simulink model "Converter2_Combined"  (R2025a)
settings: Solver=ode15s  StartTime=0.0  StopTime=10  MaxStep=1e-4  RelTol=1e-4  EnableMultiTasking=on
libraries: spsCurrentMeasurementLib x5, spsSeriesRLCBranchLib x5, spsDCVoltageSourceLib x2, slpidlib x2, spsPWMGenerator2LevelLib x2, spsMosfetLib x2, simulink x2, spsVoltageMeasurementLib x2, spsControlledCurrentSourceLib x1, spsFirstOrderFilterLib x1, spsGroundLib x1, spspowerguiLib x1
settings Model: SimulationMode=accelerator  Creator=The MathWorks, Inc.  LastModifiedBy=kaust
settings SolverCC: MaxOrder=4.0  ZeroCrossAlgorithm=Adaptive
settings DataIOCC: LimitDataPoints=on  SaveFormat=Array  SaveOutput=off  SignalLogging=off  SaveTime=off  ReturnWorkspaceOutputs=off
settings OptimizationCC: ExpressionDepthLimit=2147483647.0  LifeSpan=inf
settings DebuggingCC: UnderspecifiedInitializationDetection=Classic  MergeDetectMultiDrivingBlocksExec=none  IgnoredZcDiagnostic=none  SolverPrmCheckMsg=warning  FcnCallInpInsideContextMsg=warning  UnconnectedInputMsg=warning  UnconnectedOutputMsg=warning  UnconnectedLineMsg=warning  StateNameClashWarn=warning  SFUnexpectedBacktrackingDiag=warning  SFNoUnconditionalDefaultTransitionDiag=warning  SFExecutionAtInitializationDiag=none  ArithmeticOperatorsInVariantConditions=warning
settings HardwareCC: ProdBitPerPointer=32.0  ProdBitPerSizeT=32.0  ProdBitPerPtrDiffT=32.0  ProdLargestAtomicFloat=None  ProdIntDivRoundTo=Undefined  ProdEndianess=Unspecified  ProdWordSize=32.0  ProdHWDeviceType=32-bit Generic
settings ModelReferenceCC: EnableRefExpFcnMdlSchedulingChecks=on  PropagateSignalLabelsOutOfModel=off
settings SFSimCC: SimUseLocalCustomCode=off  CustomCodeUndefinedFunction=UseInterfaceOnly
settings RTWCC: RTWUseLocalCustomCode=off  GPUComputeCapability=3.5  DLArmComputeVersion=19.05
settings CodeAppCC: StateflowObjectComments=on
settings GRTTargetCC: TargetLangStandard=C89/C90 (ANSI)  CombineOutputUpdateFcns=off  GRTInterface=on
settings ConfigComp: CovMetricSettings=dw  CovSaveCumulativeToWorkspaceVar=on  CovSaveSingleToWorkspaceVar=on  CovExternalEMLEnable=off  CovSFcnEnable=off
settings SimscapeCC: SimscapeNormalizeSystem=off  SimscapeNominalValues={1, 'bar'; 1, 'cm^3/s'; 1, 'bar*kg/s'; 1, 'kJ/kg'; 1, 'kW'; }

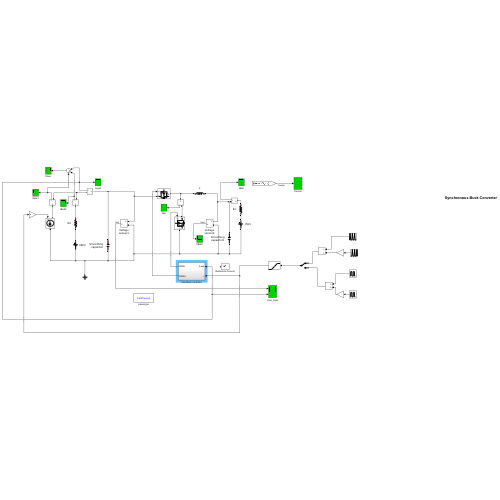
[thumbnail: Simulink's stored preview of the top-level diagram]
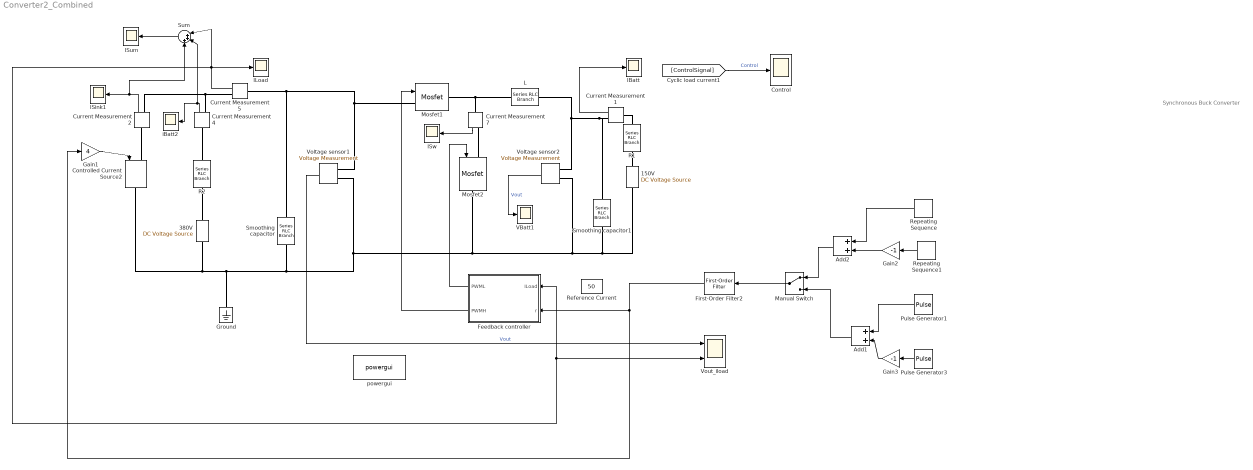
== system Converter2_Combined ==
  note: Synchronous Buck Converter
  150V : spsDCVoltageSourceLib/DC Voltage Source  Amplitude=150  Measurements=None
  380V : spsDCVoltageSourceLib/DC Voltage Source  Amplitude=380  Measurements=None
  Add1 : Sum
  Add2 : Sum
  Control : Scope
      settings: TimeSpan=0.01  ActiveDisplayYMinimum=-0.0024647053532001208  ActiveDisplayYMaximum=0.023182348178801094  DataLoggingVariableName=Control  DataLoggingSaveFormat=Array
  Controlled Current Source2 : spsControlledCurrentSourceLib/Controlled Current Source  Initialize=on  Source_Type=AC  Amplitude=0  Phase=0  Frequency=0  Measurements=None
  Current Measurement{1..2,4..5,7} (5 alike) : spsCurrentMeasurementLib/Current Measurement  PhasorSimulation=off  OutputType=Complex  PSBequivalent=0
  Feedback controller : Subsystem
  First-Order Filter2 : spsFirstOrderFilterLib/First-Order Filter  FilterType=Lowpass  Tc=5e-3  Ts=0  Initialize=off  Vac_Init=[0, 0, 60]  Vdc_Init=0  PlotResponse=off  FreqRange="[0,  200,  1]"
  Gain1 : Gain  Gain=4
  Gain2 : Gain  Gain=-1
  Gain3 : Gain  Gain=-1
  Ground : spsGroundLib/Ground  LConnTagsString=a
  IBatt : Scope
      settings: TimeSpan=0.01  ActiveDisplayYMinimum=-4410.7984256590225  ActiveDisplayYMaximum=16926.559366246598  DataLoggingVariableName=Isrc_sps1  DataLoggingSaveFormat=Array
  ILoad : Scope
      settings: TimeSpan=0.01  ActiveDisplayYMinimum=-119.68929460234355  ActiveDisplayYMaximum=1093.0850139818504  DataLoggingVariableName=Isrc_sps  DataLoggingSaveFormat=Array
  ISink1 : Scope
      settings: TimeSpan=0.01  ActiveDisplayYMinimum=-12.499999999999996  ActiveDisplayYMaximum=112.5  DataLoggingVariableName=Isrc_sps3  DataLoggingSaveFormat=Array
  ISum : Scope
      settings: TimeSpan=0.01  ActiveDisplayYMinimum=-1.7763568394002505E-14  ActiveDisplayYMaximum=1.7763568394002505E-14  DataLoggingVariableName=Isrc_sps4  DataLoggingSaveFormat=Array
  ISw : Scope
      settings: TimeSpan=0.01  ActiveDisplayYMinimum=-4410.7984256590225  ActiveDisplayYMaximum=16926.559366246598  DataLoggingVariableName=Isrc_sps6  DataLoggingSaveFormat=Array
  L : spsSeriesRLCBranchLib/Series RLC Branch  LConnTagsString=__new0  RConnTagsString=__new0  BranchType=L  Resistance=15  Inductance=1e-06  SetiL0=off  InitialCurrent=0  Capacitance=1e-6  Setx0=off  InitialVoltage=0  Measurements=None
  Manual Switch : ManualSwitch
  Mosfet1 : spsMosfetLib/Mosfet  Ron=0.1  Lon=0  Rd=0.01  Vfd=0.8  IC=0  Rs=1e5  Cs=inf  Measurements=off
  Mosfet2 : spsMosfetLib/Mosfet  Ron=0.1  Lon=0  Rd=0.01  Vfd=0.8  IC=0  Rs=1e4  Cs=inf  Measurements=off
  Pulse Generator1 : DiscretePulseGenerator  PulseType=Time based  Amplitude=50  Period=0.5  PulseWidth=50
  Pulse Generator3 : DiscretePulseGenerator  PulseType=Time based  Amplitude=50  Period=0.5  PulseWidth=50  PhaseDelay=0.25
  R1 : spsSeriesRLCBranchLib/Series RLC Branch  LConnTagsString=__new0  RConnTagsString=__new0  BranchType=R  Resistance=0.01  Inductance=1e-3  SetiL0=off  InitialCurrent=0  Capacitance=1e-6  Setx0=off  InitialVoltage=0  Measurements=None
  R2 : spsSeriesRLCBranchLib/Series RLC Branch  LConnTagsString=__new0  RConnTagsString=__new0  BranchType=R  Resistance=0.01  Inductance=1e-3  SetiL0=off  InitialCurrent=0  Capacitance=1e-6  Setx0=off  InitialVoltage=0  Measurements=None
  Reference Current : Constant  Value=50
  Repeating Sequence : simulink/Sources/Repeating Sequence  rep_seq_t=[0 0.25 0.5 0.75 1 ]  rep_seq_y=[0 50 0 0 0]
  Repeating Sequence1 : simulink/Sources/Repeating Sequence  rep_seq_t=[0 0.25 0.5 0.75 1 ]  rep_seq_y=[0 0 0 50 0]
  Smoothing capacitor : spsSeriesRLCBranchLib/Series RLC Branch  LConnTagsString=__new0  RConnTagsString=__new0  BranchType=C  Resistance=1  Inductance=1e-3  SetiL0=off  InitialCurrent=0  Capacitance=10e-3  Setx0=off  InitialVoltage=0  Measurements=None
  Smoothing capacitor1 : spsSeriesRLCBranchLib/Series RLC Branch  LConnTagsString=__new0  RConnTagsString=__new0  BranchType=C  Resistance=1  Inductance=1e-3  SetiL0=off  InitialCurrent=0  Capacitance=10e-3  Setx0=off  InitialVoltage=0  Measurements=None
  Sum : Sum  Inputs=|+++
  VBatt1 : Scope
      settings: TimeSpan=0.01  ActiveDisplayYMinimum=-4410.7984256590225  ActiveDisplayYMaximum=16926.559366246598  DataLoggingVariableName=Isrc_sps5  DataLoggingSaveFormat=Array
  Voltage sensor1 : spsVoltageMeasurementLib/Voltage Measurement  PhasorSimulation=off  OutputType=Complex  PSBequivalent=0
  Voltage sensor2 : spsVoltageMeasurementLib/Voltage Measurement  PhasorSimulation=off  OutputType=Complex  PSBequivalent=0
  Vout_iload : Scope  NumInputPorts=2
      settings: TimeSpan=0.01  ActiveDisplayYMinimum=376.83408924703053  ActiveDisplayYMaximum=382.12539978082276  DataLoggingVariableName=Vout_sps  DataLoggingSaveFormat=Array
  iBatt2 : Scope
      settings: TimeSpan=0.01  ActiveDisplayYMinimum=-212.44166562760256  ActiveDisplayYMaximum=295.23155792169746  DataLoggingVariableName=Isrc_sps2  DataLoggingSaveFormat=Array
  powergui : spspowerguiLib/powergui  Priority=1  SimulationMode=Continuous  SampleTime=50e-6  frequency=60  Iterations=50  frequencyindice=0  Pbase=100e6  ErrMax=1e-4  UnitsV=kV  UnitsW=MW  buscounter=0  FunctionMessages=off  echomessages=off  EnableUseOfTLC=off  CurrentSourceSwitches=off  DisableSnubberDevices=off  DisableRonSwitches=off  DisableVfSwitches=off  DisplayEquations=off  AutomaticDiscreteSolvers=off  SolverType=Tustin/Backward Euler (TBE)  Interpol=off  ExternalGateDelay=off  methode=off  Ts=100  x0status=blocks  SPID=on  SwTol=0  HookPort=off  NonlinearTolerance=1e-4  nMaxIteration=100  ContinueOnMaxIteration=off  RestoreLinks=warning  ResistiveCurrentMeasurement=off  Frange=[0:2:500]  Ylog=off  Xlog=on  ShowGrid=off  save=off  variable=ZData  structure=0  ZoomFFT=on  StartTime=0.0  cycles=1  DisplayStyle=1  fundamental=60  FreqAxis=off  MaxFrequency=1000  frequencyindicesteady=1  RmsSteady=1  display=off
  wires:
  Feedback controller/1(PWML) -> Mosfet2/1
  [ControlSignal] -> Control/1  "Control"
  Current Measurement5/1 -> Sum/1, ILoad/1, Feedback controller/1(ILoad), Vout_iload/2
  Feedback controller/2(PWMH) -> Mosfet1/1
  Voltage sensor1/1 -> Vout_iload/1  "Vout"
  Current Measurement1/1 -> IBatt/1
  Current Measurement4/1 -> iBatt2/1, Sum/2
  Current Measurement2/1 -> Sum/3, ISink1/1
  Sum/1 -> ISum/1
  Voltage sensor2/1 -> VBatt1/1  "Vout"
  Current Measurement7/1 -> ISw/1
  First-Order Filter2/1 -> Feedback controller/2(r), Gain1/1
  Gain1/1 -> Controlled Current Source2/1
  Repeating Sequence/1 -> Add2/1
  Repeating Sequence1/1 -> Gain2/1
  Gain2/1 -> Add2/2
  Add2/1 -> Manual Switch/1
  Manual Switch/1 -> First-Order Filter2/1
  Gain3/1 -> Add1/2
  Add1/1 -> Manual Switch/2
  Pulse Generator1/1 -> Add1/1
  Pulse Generator3/1 -> Gain3/1
  connections:
  Mosfet2/RConn1 -- Smoothing capacitor/RConn1 -- Controlled Current Source2/RConn1 -- 380V/LConn1 -- Ground/LConn1 -- Voltage sensor1/LConn2 -- Smoothing capacitor1/RConn1 -- 150V/LConn1 -- Voltage sensor2/LConn2
  L/RConn1 -- Smoothing capacitor1/LConn1 -- Current Measurement1/RConn1 -- Voltage sensor2/LConn1
  L/LConn1 -- Current Measurement7/LConn1 -- Mosfet1/RConn1
  Smoothing capacitor/LConn1 -- Voltage sensor1/LConn1 -- Mosfet1/LConn1 -- Current Measurement5/LConn1
  150V/RConn1 -- R1/RConn1
  Current Measurement5/RConn1 -- Current Measurement2/RConn1 -- Current Measurement4/RConn1
  Current Measurement2/LConn1 -- Controlled Current Source2/LConn1
  380V/RConn1 -- R2/RConn1
  Current Measurement4/LConn1 -- R2/LConn1
  R1/LConn1 -- Current Measurement1/LConn1
  Current Measurement7/RConn1 -- Mosfet2/LConn1

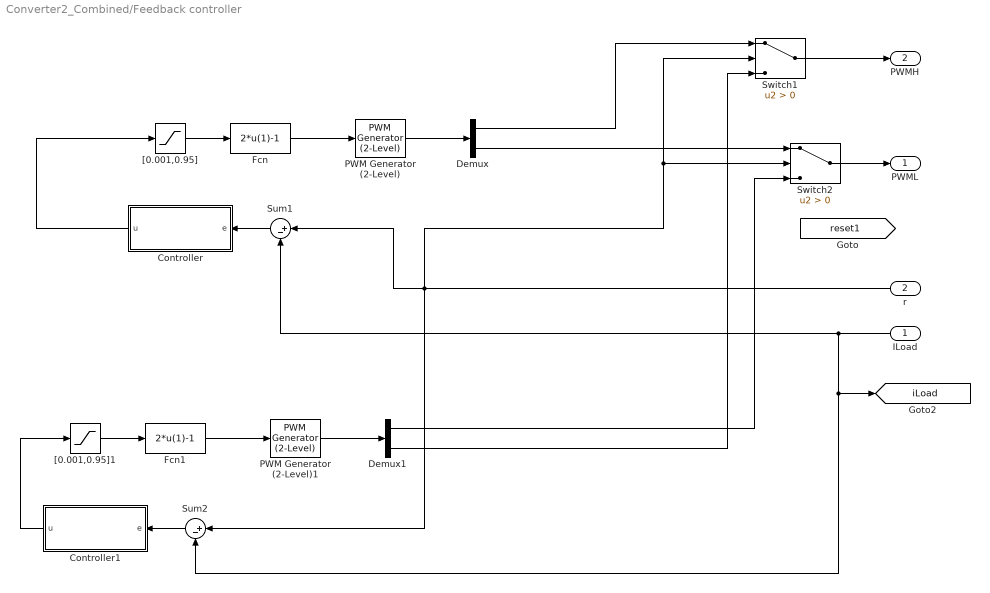
== system Converter2_Combined/Feedback controller ==
  ILoad : Inport
  r : Inport  Port=2
  Controller : Subsystem  Variant=on  VariantControlMode=label  LabelModeActiveChoice=Variant1
      settings: AttributesFormatString=%<BlockChoice>
  Controller1 : Subsystem  Variant=on  VariantControlMode=label  LabelModeActiveChoice=Variant1
      settings: AttributesFormatString=%<BlockChoice>
  Demux : Demux  Outputs=2
  Demux1 : Demux  Outputs=2
  Fcn : Fcn  Expr=2*u(1)-1
  Fcn1 : Fcn  Expr=2*u(1)-1
  PWM Generator (2-Level) : spsPWMGenerator2LevelLib/PWM Generator (2-Level)  ModulatorType=Single-phase half-bridge (2 pulses)  ModulatorMode=Unsynchronized  Fc=50000  Pc=90  nF=27  MinMax="[ -1  1 ]"  SamplingTechnique=Natural  ModulatingSignals=off  m=0.8  Freq=60  Phase=0  Ts=0  ShowCarrierOutport=off
  PWM Generator (2-Level)1 : spsPWMGenerator2LevelLib/PWM Generator (2-Level)  ModulatorType=Single-phase half-bridge (2 pulses)  ModulatorMode=Unsynchronized  Fc=50000  Pc=90  nF=27  MinMax="[ -1  1 ]"  SamplingTechnique=Natural  ModulatingSignals=off  m=0.8  Freq=60  Phase=0  Ts=0  ShowCarrierOutport=off
  Sum1 : Sum  Inputs=|+-  InputSameDT=on  SaturateOnIntegerOverflow=on  OutDataTypeStr=Inherit: Same as first input
  Sum2 : Sum  Inputs=|+-  InputSameDT=on  SaturateOnIntegerOverflow=on  OutDataTypeStr=Inherit: Same as first input
  Switch1 : Switch  Criteria=u2 > Threshold  SaturateOnIntegerOverflow=off  InputSameDT=off
  Switch2 : Switch  Criteria=u2 > Threshold  SaturateOnIntegerOverflow=off  InputSameDT=off
  "[0.001,0.95]" : Saturate  UpperLimit=0.95  LowerLimit=0.0001
  "[0.001,0.95]1" : Saturate  UpperLimit=0.95  LowerLimit=0.0001
  PWML : Outport  VectorParamsAs1DForOutWhenUnconnected=off
  PWMH : Outport  Port=2  VectorParamsAs1DForOutWhenUnconnected=off
  tag scope: iLoad=global, reset1=global
  wires:
  Controller/1(u) -> "[0.001,0.95]"/1
  PWM Generator (2-Level)/1 -> Demux/1
  Demux/1 -> Switch1/1
  Demux/2 -> Switch2/1
  Sum1/1 -> Controller/1(e)
  "[0.001,0.95]"/1 -> Fcn/1
  Fcn/1 -> PWM Generator (2-Level)/1
  PWM Generator (2-Level)1/1 -> Demux1/1
  r/1 -> Switch2/2, Switch1/2, Sum2/1, Sum1/1
  Fcn1/1 -> PWM Generator (2-Level)1/1
  "[0.001,0.95]1"/1 -> Fcn1/1
  Controller1/1(u) -> "[0.001,0.95]1"/1
  Sum2/1 -> Controller1/1(e)
  Demux1/2 -> Switch1/3
  ILoad/1 -> [iLoad], Sum2/2, Sum1/2
  Demux1/1 -> Switch2/3
  Switch1/1 -> PWMH/1
  Switch2/1 -> PWML/1

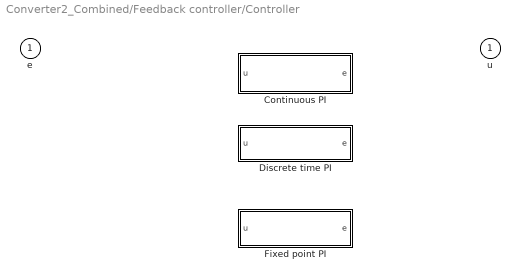
== system Converter2_Combined/Feedback controller/Controller ==
  e : Inport
  Continuous PI : Subsystem  VariantControl=Variant1
  Discrete time PI : Subsystem  VariantControl=Variant2
  Fixed point PI : Subsystem  MinMaxOverflowLogging=MinMaxAndOverflow  VariantControl=Variant3
  u : Outport  VectorParamsAs1DForOutWhenUnconnected=off

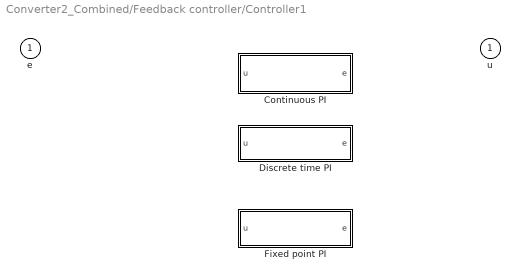
== system Converter2_Combined/Feedback controller/Controller1 ==
  e : Inport
  Continuous PI : Subsystem  VariantControl=Variant1
  Discrete time PI : Subsystem  VariantControl=Variant2
  Fixed point PI : Subsystem  MinMaxOverflowLogging=MinMaxAndOverflow  VariantControl=Variant3
  u : Outport  VectorParamsAs1DForOutWhenUnconnected=off

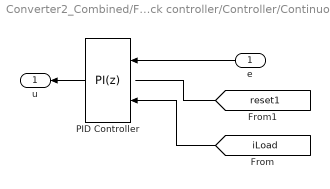
== system Converter2_Combined/Feedback controller/Controller/Continuous PI ==
  e : Inport
  PID Controller : slpidlib/PID Controller  Controller=PI  Form=Parallel  TimeDomain=Discrete-time  UseExternalTs=off  SampleTime=-1  IntegratorMethod=Forward Euler  FilterMethod=Forward Euler  ControllerParametersSource=internal  P=0.01  I=1  UseKiTs=off  D=0.01  UseExternalDerivativeSource=off  N=100  UseFilter=on  TunerSelectOption=Transfer Function Based (PID Tuner App)  InitialConditionSource=internal  InitialConditionForIntegrator=0  InitialConditionForFilter=0  DifferentiatorICPrevScaledInput=0  ExternalReset=none  TrackingMode=on  Kt=0.01  LimitOutput=on  SatLimitsSource=internal  UpperSaturationLimit=1  LowerSaturationLimit=0  LinearizeAsGain=on  AntiWindupMode=clamping  Kb=0.05  LimitIntegrator=off  UpperIntegratorSaturationLimit=inf  LowerIntegratorSaturationLimit=-inf  POutMin=[]  POutMax=[]  IOutMin=[]  IOutMax=[]  DOutMin=[]  DOutMax=[]  NOutMin=[]  NOutMax=[]  SumOutMin=[]  SumOutMax=[]  SaturationOutMin=[]  SaturationOutMax=[]  PParamMin=[]  PParamMax=[]  IParamMin=[]  IParamMax=[]  DParamMin=[]  DParamMax=[]  NParamMin=[]  NParamMax=[]  KbParamMin=[]  KbParamMax=[]  KtParamMin=[]  KtParamMax=[]  KbOutMin=[]  KbOutMax=[]  KtOutMin=[]  KtOutMax=[]  IntegratorOutMin=[]  IntegratorOutMax=[]  FilterOutMin=[]  FilterOutMax=[]  SumI1OutMin=[]  SumI1OutMax=[]  SumI2OutMin=[]  SumI2OutMax=[]  SumI3OutMin=[]  SumI3OutMax=[]  SumI4OutMin=[]  SumI4OutMax=[]  SumDOutMin=[]  SumDOutMax=[]  DifferentiatorOutMin=[]  DifferentiatorOutMax=[]  FilterDiffOutCoefMin=[]  FilterDiffOutCoefMax=[]  ReciprocalOutMin=[]  ReciprocalOutMax=[]  SumDenOutMin=[]  SumDenOutMax=[]  SumNumOutMin=[]  SumNumOutMax=[]  DivideOutMin=[]  DivideOutMax=[]  UdiffTsProdOutMin=[]  UdiffTsProdOutMax=[]  NTsProdOutMin=[]  NTsProdOutMax=[]  UintegralTsProdOutMin=[]  UintegralTsProdOutMax=[]  UngainTsProdOutMin=[]  UngainTsProdOutMax=[]  ClampingZeroOutDataTypeStr=Inherit: Inherit via back propagation  ClampingZeroOutMin=[]  ClampingZeroOutMax=[]  FilterDenConstantOutDataTypeStr=Inherit: Inherit via back propagation  FilterDenConstantOutMin=[]  FilterDenConstantOutMax=[]  PCopyOutDataTypeStr=Inherit: Inherit via back propagation  PCopyOutMin=[]  PCopyOutMax=[]  NCopyOutDataTypeStr=Inherit: Inherit via back propagation  NCopyOutMin=[]  NCopyOutMax=[]  IntegratorContinuousStateAttributes=''  IntegratorStateMustResolveToSignalObject=off  IntegratorRTWStateStorageClass=Auto  FilterContinuousStateAttributes=''  FilterStateMustResolveToSignalObject=off  FilterRTWStateStorageClass=Auto  ParallelPVariant=InternalParameters  IdealPVariant=Disabled  IVariant=InternalParameters  DVariant=Disabled  IntegratorVariant=Discrete  SatVariant=Enabled  AWVariant=DiscClampingParallel  PCopyVariant=Disabled  TRVariant=Enabled  FdbkBlocksVariant=Forward  IdealPFdbkVariant=Disabled  SatFdbkVariant=Disabled  DerivativeFilterVariant=Disabled  NVariant=Disabled  NCopyVariant=Disabled_SignalSpec  FilterICVariant=Disabled  IntegratorICVariant=InternalICs  ExternalResetVariant=Disabled  TRSumVariant=TrackingMode  SumFdbkVariant=Disabled  SumVariant=Sum_PI  TsampFilterVariant=InternalTs  TsampNgainVariant=Passthrough  TsampIntegralVariant=Disabled_SignalSpec  ExternalSaturationOutDataTypeStr=Inherit: Same as second input  DerivativeSourceVariant=Disabled  PreIntVariant=InternalPreInt
  u : Outport  VectorParamsAs1DForOutWhenUnconnected=off
  wires:
  [iLoad] -> PID Controller/2
  PID Controller/1 -> u/1
  e/1 -> PID Controller/1
  [reset1] -> ?

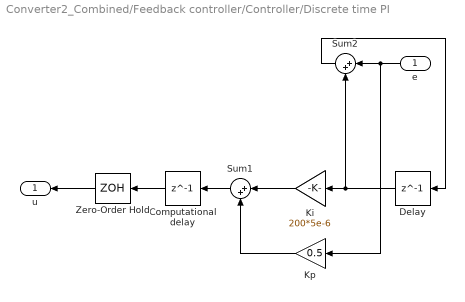
== system Converter2_Combined/Feedback controller/Controller/Discrete time PI ==
  e : Inport
  Computational delay : Delay  DelayLength=1  SampleTime=5e-6
  Delay : Delay  DelayLength=1  SampleTime=5e-6
  Ki : Gain  Gain=200*5e-6
  Kp : Gain  Gain=0.5
  Sum1 : Sum  Inputs=|++  InputSameDT=on  SaturateOnIntegerOverflow=on  OutDataTypeStr=Inherit: Same as first input
  Sum2 : Sum  Inputs=|++  InputSameDT=on  SaturateOnIntegerOverflow=on  OutDataTypeStr=Inherit: Same as first input
  Zero-Order Hold : ZeroOrderHold  SampleTime=5e-6
  u : Outport  VectorParamsAs1DForOutWhenUnconnected=off
  wires:
  Ki/1 -> Sum1/1
  Sum2/1 -> Delay/1
  Delay/1 -> Ki/1, Sum2/2
  Kp/1 -> Sum1/2
  Sum1/1 -> Computational delay/1
  e/1 -> Kp/1, Sum2/1
  Zero-Order Hold/1 -> u/1
  Computational delay/1 -> Zero-Order Hold/1

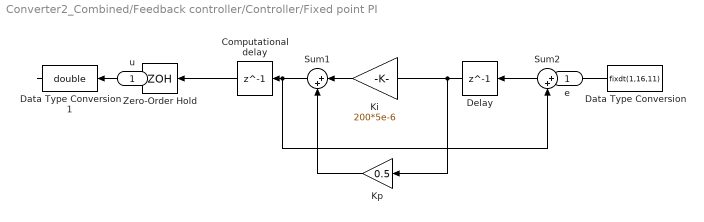
== system Converter2_Combined/Feedback controller/Controller/Fixed point PI ==
  e : Inport
  Computational delay : Delay  DelayLength=1  SampleTime=5e-6
  Data Type Conversion : DataTypeConversion  OutDataTypeStr=fixdt(1,16,11)  RndMeth=Nearest  SaturateOnIntegerOverflow=off
  Data Type Conversion1 : DataTypeConversion  OutDataTypeStr=double  RndMeth=Nearest  SaturateOnIntegerOverflow=off
  Delay : Delay  DelayLength=1  SampleTime=5e-6
  Ki : Gain  Gain=200*5e-6  OutDataTypeStr=fixdt(1,16,13)  RndMeth=Nearest
  Kp : Gain  Gain=0.5  OutDataTypeStr=fixdt(1,16,9)  RndMeth=Nearest
  Sum1 : Sum  Inputs=|++  SaturateOnIntegerOverflow=on
  Sum2 : Sum  Inputs=|++  InputSameDT=on  SaturateOnIntegerOverflow=on  OutDataTypeStr=Inherit: Same as first input
  Zero-Order Hold : ZeroOrderHold  SampleTime=5e-6
  u : Outport  VectorParamsAs1DForOutWhenUnconnected=off
  wires:
  Ki/1 -> Sum1/1
  Data Type Conversion1/1 -> u/1
  Data Type Conversion/1 -> Sum2/1, Kp/1
  Sum1/1 -> Computational delay/1
  Kp/1 -> Sum1/2
  e/1 -> Data Type Conversion/1
  Delay/1 -> Ki/1, Sum2/2
  Sum2/1 -> Delay/1
  Computational delay/1 -> Zero-Order Hold/1
  Zero-Order Hold/1 -> Data Type Conversion1/1

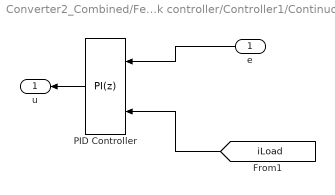
== system Converter2_Combined/Feedback controller/Controller1/Continuous PI ==
  e : Inport
  PID Controller : slpidlib/PID Controller  Controller=PI  Form=Parallel  TimeDomain=Discrete-time  UseExternalTs=off  SampleTime=-1  IntegratorMethod=Forward Euler  FilterMethod=Forward Euler  ControllerParametersSource=internal  P=0.0025  I=1  UseKiTs=off  D=1  UseExternalDerivativeSource=off  N=100  UseFilter=on  TunerSelectOption=Transfer Function Based (PID Tuner App)  InitialConditionSource=internal  InitialConditionForIntegrator=0  InitialConditionForFilter=0  DifferentiatorICPrevScaledInput=0  ExternalReset=none  TrackingMode=on  Kt=0.01  LimitOutput=on  SatLimitsSource=internal  UpperSaturationLimit=1  LowerSaturationLimit=0  LinearizeAsGain=on  AntiWindupMode=clamping  Kb=0.05  LimitIntegrator=off  UpperIntegratorSaturationLimit=inf  LowerIntegratorSaturationLimit=-inf  POutMin=[]  POutMax=[]  IOutMin=[]  IOutMax=[]  DOutMin=[]  DOutMax=[]  NOutMin=[]  NOutMax=[]  SumOutMin=[]  SumOutMax=[]  SaturationOutMin=[]  SaturationOutMax=[]  PParamMin=[]  PParamMax=[]  IParamMin=[]  IParamMax=[]  DParamMin=[]  DParamMax=[]  NParamMin=[]  NParamMax=[]  KbParamMin=[]  KbParamMax=[]  KtParamMin=[]  KtParamMax=[]  KbOutMin=[]  KbOutMax=[]  KtOutMin=[]  KtOutMax=[]  IntegratorOutMin=[]  IntegratorOutMax=[]  FilterOutMin=[]  FilterOutMax=[]  SumI1OutMin=[]  SumI1OutMax=[]  SumI2OutMin=[]  SumI2OutMax=[]  SumI3OutMin=[]  SumI3OutMax=[]  SumI4OutMin=[]  SumI4OutMax=[]  SumDOutMin=[]  SumDOutMax=[]  DifferentiatorOutMin=[]  DifferentiatorOutMax=[]  FilterDiffOutCoefMin=[]  FilterDiffOutCoefMax=[]  ReciprocalOutMin=[]  ReciprocalOutMax=[]  SumDenOutMin=[]  SumDenOutMax=[]  SumNumOutMin=[]  SumNumOutMax=[]  DivideOutMin=[]  DivideOutMax=[]  UdiffTsProdOutMin=[]  UdiffTsProdOutMax=[]  NTsProdOutMin=[]  NTsProdOutMax=[]  UintegralTsProdOutMin=[]  UintegralTsProdOutMax=[]  UngainTsProdOutMin=[]  UngainTsProdOutMax=[]  ClampingZeroOutDataTypeStr=Inherit: Inherit via back propagation  ClampingZeroOutMin=[]  ClampingZeroOutMax=[]  FilterDenConstantOutDataTypeStr=Inherit: Inherit via back propagation  FilterDenConstantOutMin=[]  FilterDenConstantOutMax=[]  PCopyOutDataTypeStr=Inherit: Inherit via back propagation  PCopyOutMin=[]  PCopyOutMax=[]  NCopyOutDataTypeStr=Inherit: Inherit via back propagation  NCopyOutMin=[]  NCopyOutMax=[]  IntegratorContinuousStateAttributes=''  IntegratorStateMustResolveToSignalObject=off  IntegratorRTWStateStorageClass=Auto  FilterContinuousStateAttributes=''  FilterStateMustResolveToSignalObject=off  FilterRTWStateStorageClass=Auto  ParallelPVariant=InternalParameters  IdealPVariant=Disabled  IVariant=InternalParameters  DVariant=Disabled  IntegratorVariant=Discrete  SatVariant=Enabled  AWVariant=DiscClampingParallel  PCopyVariant=Disabled  TRVariant=Enabled  FdbkBlocksVariant=Forward  IdealPFdbkVariant=Disabled  SatFdbkVariant=Disabled  DerivativeFilterVariant=Disabled  NVariant=Disabled  NCopyVariant=Disabled_SignalSpec  FilterICVariant=Disabled  IntegratorICVariant=InternalICs  ExternalResetVariant=Disabled  TRSumVariant=TrackingMode  SumFdbkVariant=Disabled  SumVariant=Sum_PI  TsampFilterVariant=InternalTs  TsampNgainVariant=Passthrough  TsampIntegralVariant=Disabled_SignalSpec  ExternalSaturationOutDataTypeStr=Inherit: Same as second input  DerivativeSourceVariant=Disabled  PreIntVariant=InternalPreInt
  u : Outport  VectorParamsAs1DForOutWhenUnconnected=off
  wires:
  [iLoad] -> PID Controller/2
  PID Controller/1 -> u/1
  e/1 -> PID Controller/1

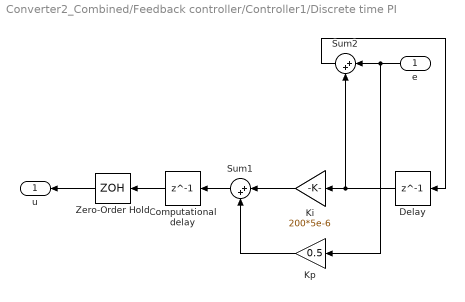
== system Converter2_Combined/Feedback controller/Controller1/Discrete time PI ==
  e : Inport
  Computational delay : Delay  DelayLength=1  SampleTime=5e-6
  Delay : Delay  DelayLength=1  SampleTime=5e-6
  Ki : Gain  Gain=200*5e-6
  Kp : Gain  Gain=0.5
  Sum1 : Sum  Inputs=|++  InputSameDT=on  SaturateOnIntegerOverflow=on  OutDataTypeStr=Inherit: Same as first input
  Sum2 : Sum  Inputs=|++  InputSameDT=on  SaturateOnIntegerOverflow=on  OutDataTypeStr=Inherit: Same as first input
  Zero-Order Hold : ZeroOrderHold  SampleTime=5e-6
  u : Outport  VectorParamsAs1DForOutWhenUnconnected=off
  wires:
  Ki/1 -> Sum1/1
  Sum2/1 -> Delay/1
  Delay/1 -> Ki/1, Sum2/2
  Kp/1 -> Sum1/2
  Sum1/1 -> Computational delay/1
  e/1 -> Kp/1, Sum2/1
  Zero-Order Hold/1 -> u/1
  Computational delay/1 -> Zero-Order Hold/1

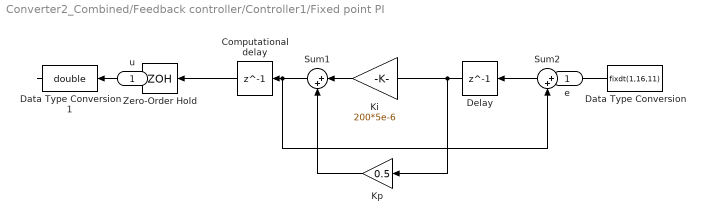
== system Converter2_Combined/Feedback controller/Controller1/Fixed point PI ==
  e : Inport
  Computational delay : Delay  DelayLength=1  SampleTime=5e-6
  Data Type Conversion : DataTypeConversion  OutDataTypeStr=fixdt(1,16,11)  RndMeth=Nearest  SaturateOnIntegerOverflow=off
  Data Type Conversion1 : DataTypeConversion  OutDataTypeStr=double  RndMeth=Nearest  SaturateOnIntegerOverflow=off
  Delay : Delay  DelayLength=1  SampleTime=5e-6
  Ki : Gain  Gain=200*5e-6  OutDataTypeStr=fixdt(1,16,13)  RndMeth=Nearest
  Kp : Gain  Gain=0.5  OutDataTypeStr=fixdt(1,16,9)  RndMeth=Nearest
  Sum1 : Sum  Inputs=|++  SaturateOnIntegerOverflow=on
  Sum2 : Sum  Inputs=|++  InputSameDT=on  SaturateOnIntegerOverflow=on  OutDataTypeStr=Inherit: Same as first input
  Zero-Order Hold : ZeroOrderHold  SampleTime=5e-6
  u : Outport  VectorParamsAs1DForOutWhenUnconnected=off
  wires:
  Ki/1 -> Sum1/1
  Data Type Conversion1/1 -> u/1
  Data Type Conversion/1 -> Sum2/1, Kp/1
  Sum1/1 -> Computational delay/1
  Kp/1 -> Sum1/2
  e/1 -> Data Type Conversion/1
  Delay/1 -> Ki/1, Sum2/2
  Sum2/1 -> Delay/1
  Computational delay/1 -> Zero-Order Hold/1
  Zero-Order Hold/1 -> Data Type Conversion1/1
